simulink model "simpowersystems_simple_phasor_source"  (Simulink 8.1)
settings: Solver=FixedStepDiscrete  StartTime=0.0  StopTime=inf  FixedStep=1  MaxStep=1/60  RelTol=1e-3
InitFcn:
  | Ts = 1e-5;
undefined symbols (not defined in the file): j
libraries: powerlib x9, powerlib_extras x3, simulink x2
settings Model: Creator=sfrank1  LastModifiedBy=bjohnson

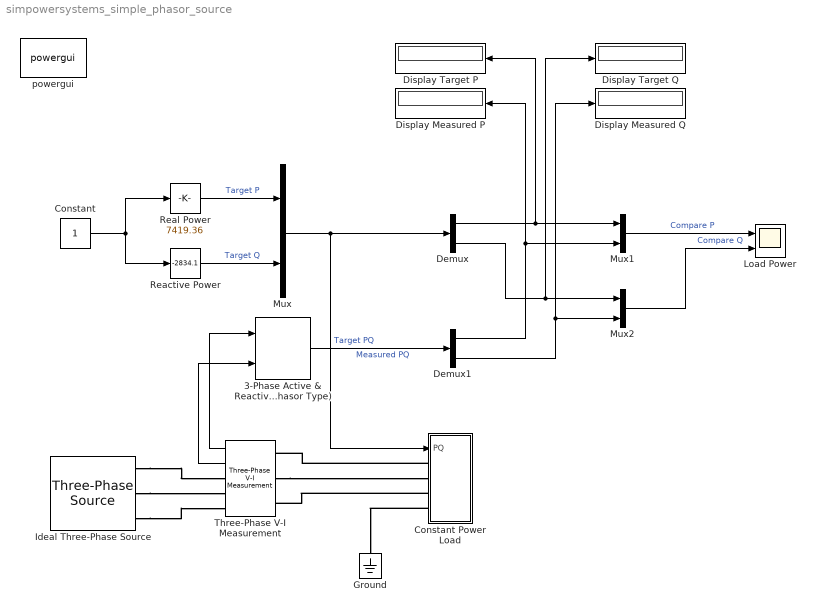
== system simpowersystems_simple_phasor_source ==
  3-Phase Active & Reactive Power (Phasor Type) : powerlib_extras/Phasor Library/3-Phase Active & Reactive Power (Phasor Type)
  Constant : Constant
  Constant Power Load : Subsystem  mask(Constant Power Load){VNom=480, fNom=60}
      mask prompts: VNom "Nominal line-to-line voltage (VRMS)"; fNom "Nominal frequency (Hz)"
      mask help: Implements a controllable constant power load, where VI* = P + jQ (in per-unit).
      mask Help: Implements a controllable constant power load, where VI* = P + jQ (in per-unit).
  Demux : Demux  Outputs=2
  Demux1 : Demux  Outputs=2
  Display Measured P : Display
  Display Measured Q : Display
  Display Target P : Display
  Display Target Q : Display
  Ground : powerlib/Elements/Ground  LConnTagsString=a
  Ideal Three-Phase Source : powerlib/Electrical Sources/Three-Phase Source  Voltage=480  PhaseAngle=0  Frequency=60  InternalConnection=Yg  SpecifyImpedance=on  Resistance=0  Inductance=0  ShortCircuitLevel=1e6  BaseVoltage=480  XRratio=1  BusType=swing  Pref=0  Qref=0  Qmin=-inf  Qmax=inf
  Load Power : Scope  NumInputPorts=2
      settings: TickLabels=on  YMin=7419.36~-2834.1  YMax=7419.36~-2834.1
  Mux : Mux  Inputs=2
  Mux1 : Mux  Inputs=2
  Mux2 : Mux  Inputs=2
  Reactive Power : simulink/Math Operations/Slider Gain  low=-5000  gain=-2834.1  high=5000
  Real Power : simulink/Math Operations/Slider Gain  low=0  gain=7419.36  high=10000
  Three-Phase V-I Measurement : powerlib/Measurements/Three-Phase V-I Measurement  VoltageMeasurement=phase-to-ground  SetLabelV=off  LabelV=Vabc  Vpu=off  VpuLL=off  CurrentMeasurement=yes  SetLabelI=off  LabelI=Iabc  Ipu=off  Pbase=100e6  Vbase=500e3  OutputType=Complex  PhasorSimulation=on  PSBequivalent=0
  powergui : powerlib/powergui  Priority=1  SimulationMode=Phasor  SolverType=Tustin  SampleTime=50e-6  frequency=60  SPID=off  DisableSnubberDevices=off  DisableRonSwitches=off  DisableVfSwitches=off  SwTol=0  Interpol=off  DisplayEquations=off  frequencyindice=60  Pbase=100e3  ErrMax=1e-4  Iterations=50  UnitsV=kV  UnitsW=MW  FunctionMessages=off  echomessages=off  HookPort=off  EnableUseOfTLC=off  x0status=blocks  RestoreLinks=warning  ResistiveCurrentMeasurement=off  Frange=[0:2:500]  Ylog=off  Xlog=on  ShowGrid=off  save=off  variable=ZData  ZoomFFT=off  StartTime=0.0  cycles=1  DisplayStyle=1  fundamental=60  FreqAxis=off  MaxFrequency=1000  frequencyindicesteady=1  RmsSteady=1  display=off  Ts=0  methode=off
  wires:
  Constant/1 -> Reactive Power/1, Real Power/1
  Real Power/1 -> Mux/1  "Target P"
  Mux/1 -> Constant Power Load/1(PQ), Demux/1  "Target PQ"
  Three-Phase V-I Measurement/1 -> 3-Phase Active & Reactive Power (Phasor Type)/1
  Three-Phase V-I Measurement/2 -> 3-Phase Active & Reactive Power (Phasor Type)/2
  Reactive Power/1 -> Mux/2  "Target Q"
  3-Phase Active & Reactive Power (Phasor Type)/1 -> Demux1/1  "Measured PQ"
  Mux1/1 -> Load Power/1  "Compare P"
  Mux2/1 -> Load Power/2  "Compare Q"
  Demux/1 -> Mux1/1, Display Target P/1
  Demux1/1 -> Display Measured P/1, Mux1/2
  Demux/2 -> Mux2/1, Display Target Q/1
  Demux1/2 -> Mux2/2, Display Measured Q/1
  connections:
  Constant Power Load/LConn3 -- Three-Phase V-I Measurement/LConn3
  Three-Phase V-I Measurement/LConn2 -- Constant Power Load/LConn2
  Constant Power Load/LConn1 -- Three-Phase V-I Measurement/LConn1
  Constant Power Load/LConn4 -- Ground/LConn1
  Ideal Three-Phase Source/RConn2 -- Three-Phase V-I Measurement/RConn2
  Ideal Three-Phase Source/RConn1 -- Three-Phase V-I Measurement/RConn1
  Ideal Three-Phase Source/RConn3 -- Three-Phase V-I Measurement/RConn3

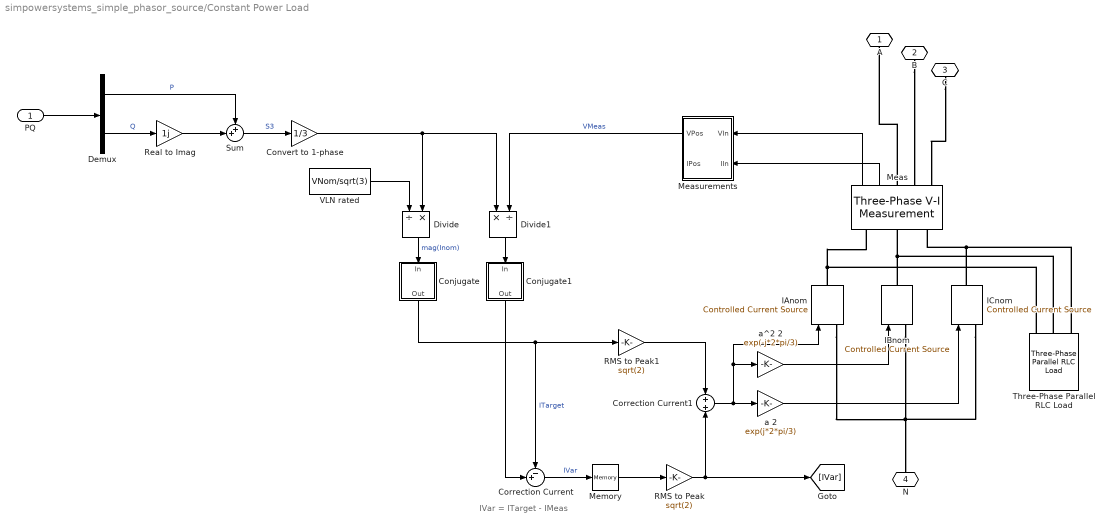
== system simpowersystems_simple_phasor_source/Constant Power Load ==
  note: IVar = ITarget - IMeas
  PQ : Inport  PortDimensions=2
  Conjugate : Subsystem
  Conjugate1 : Subsystem
  Convert to 1-phase : Gain  Gain=1/3
  Correction Current : Sum  Inputs=-+|
  Correction Current1 : Sum
  Demux : Demux  Outputs=2
  Divide : Product  Inputs=/*
  Divide1 : Product  Inputs=*/
  IAnom : powerlib/Electrical Sources/Controlled Current Source  Initialize=off  Source_Type=AC  Amplitude=0  Phase=0  Frequency=0  Measurements=Current
  IBnom : powerlib/Electrical Sources/Controlled Current Source  Initialize=off  Source_Type=AC  Amplitude=0  Phase=0  Frequency=0  Measurements=Current
  ICnom : powerlib/Electrical Sources/Controlled Current Source  Initialize=off  Source_Type=AC  Amplitude=0  Phase=0  Frequency=0  Measurements=Current
  Meas : powerlib/Measurements/Three-Phase V-I Measurement  VoltageMeasurement=phase-to-ground  SetLabelV=off  LabelV=Vabc  Vpu=off  VpuLL=off  CurrentMeasurement=yes  SetLabelI=off  LabelI=Iabc  Ipu=off  Pbase=100e6  Vbase=VNom  OutputType=Complex  PhasorSimulation=on  PSBequivalent=0
  Measurements : Subsystem
  Memory : Memory
  RMS to Peak : Gain  Gain=sqrt(2)
  RMS to Peak1 : Gain  Gain=sqrt(2)
  Real to Imag : Gain  Gain=1j
  Sum : Sum  Inputs=++|
  Three-Phase Parallel RLC Load : powerlib/Elements/Three-Phase Parallel RLC Load  LConnTagsString=A|B|C  Configuration=Y (grounded)  NominalVoltage=480  NominalFrequency=60  ActivePower=1e-9  InductivePower=0  CapacitivePower=0  Measurements=None  LoadType=constant Z
  VLN rated : Constant  Value=VNom/sqrt(3)
  a 2 : Gain  Gain=exp(j*2*pi/3)
  a^2 2 : Gain  Gain=exp(-j*2*pi/3)
  A : PMIOPort  Port=1  Side=Left
  B : PMIOPort  Port=2  Side=Left
  C : PMIOPort  Port=3  Side=Left
  N : PMIOPort  Port=4  Side=Left
  wires:
  PQ/1 -> Demux/1
  Demux/2 -> Real to Imag/1  "Q"
  Demux/1 -> Sum/1  "P"
  Real to Imag/1 -> Sum/2
  Sum/1 -> Convert to 1-phase/1  "S3"
  Convert to 1-phase/1 -> Divide/2, Divide1/1
  Divide/1 -> Conjugate/1(In)  "mag(Inom)"
  Correction Current/1 -> Memory/1  "IVar"
  Conjugate/1(Out) -> Correction Current/1, RMS to Peak1/1  "ITarget"
  RMS to Peak/1 -> [IVar], Correction Current1/2
  Memory/1 -> RMS to Peak/1
  VLN rated/1 -> Divide/1
  a 2/1 -> ICnom/1
  a^2 2/1 -> IBnom/1
  Meas/1 -> Measurements/1(VIn)
  Meas/2 -> Measurements/2(IIn)
  Measurements/1(VPos) -> Divide1/2  "VMeas"
  Divide1/1 -> Conjugate1/1(In)
  Conjugate1/1(Out) -> Correction Current/2
  Correction Current1/1 -> a^2 2/1, IAnom/1, a 2/1
  RMS to Peak1/1 -> Correction Current1/1
  connections:
  Meas/RConn1 -- A/RConn1
  B/RConn1 -- Meas/RConn2
  C/RConn1 -- Meas/RConn3
  IAnom/RConn1 -- Three-Phase Parallel RLC Load/LConn1 -- Meas/LConn1
  IBnom/RConn1 -- Three-Phase Parallel RLC Load/LConn2 -- Meas/LConn2
  ICnom/RConn1 -- Three-Phase Parallel RLC Load/LConn3 -- Meas/LConn3
  IBnom/LConn1 -- ICnom/LConn1 -- N/RConn1 -- IAnom/LConn1

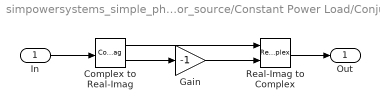
== system simpowersystems_simple_phasor_source/Constant Power Load/Conjugate ==
  In : Inport
  Complex to Real-Imag : ComplexToRealImag
  Gain : Gain  Gain=-1
  Real-Imag to Complex : RealImagToComplex
  Out : Outport
  wires:
  In/1 -> Complex to Real-Imag/1
  Complex to Real-Imag/1 -> Real-Imag to Complex/1
  Complex to Real-Imag/2 -> Gain/1
  Gain/1 -> Real-Imag to Complex/2
  Real-Imag to Complex/1 -> Out/1

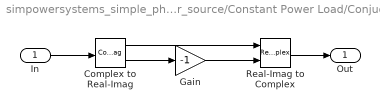
== system simpowersystems_simple_phasor_source/Constant Power Load/Conjugate1 ==
  In : Inport
  Complex to Real-Imag : ComplexToRealImag
  Gain : Gain  Gain=-1
  Real-Imag to Complex : RealImagToComplex
  Out : Outport
  wires:
  Real-Imag to Complex/1 -> Out/1
  Gain/1 -> Real-Imag to Complex/2
  Complex to Real-Imag/2 -> Gain/1
  Complex to Real-Imag/1 -> Real-Imag to Complex/1
  In/1 -> Complex to Real-Imag/1

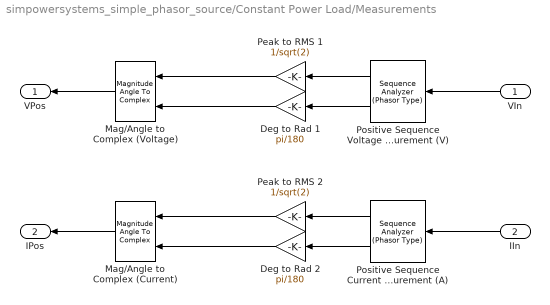
== system simpowersystems_simple_phasor_source/Constant Power Load/Measurements ==
  VIn : Inport
  IIn : Inport  Port=2
  Deg to Rad 1 : Gain  Gain=pi/180
  Deg to Rad 2 : Gain  Gain=pi/180
  Mag/Angle to Complex (Current) : MagnitudeAngleToComplex
  Mag/Angle to Complex (Voltage) : MagnitudeAngleToComplex
  Peak to RMS 1 : Gain  Gain=1/sqrt(2)
  Peak to RMS 2 : Gain  Gain=1/sqrt(2)
  Positive Sequence Current Measurement (A) : powerlib_extras/Phasor Library/Sequence Analyzer (Phasor Type)  seq=Positive
  Positive Sequence Voltage Measurement (V) : powerlib_extras/Phasor Library/Sequence Analyzer (Phasor Type)  seq=Positive
  VPos : Outport
  IPos : Outport  Port=2
  wires:
  Positive Sequence Voltage Measurement (V)/1 -> Peak to RMS 1/1
  Positive Sequence Current Measurement (A)/1 -> Peak to RMS 2/1
  Positive Sequence Current Measurement (A)/2 -> Deg to Rad 2/1
  Peak to RMS 1/1 -> Mag/Angle to Complex (Voltage)/1
  VIn/1 -> Positive Sequence Voltage Measurement (V)/1
  IIn/1 -> Positive Sequence Current Measurement (A)/1
  Mag/Angle to Complex (Voltage)/1 -> VPos/1
  Mag/Angle to Complex (Current)/1 -> IPos/1
  Peak to RMS 2/1 -> Mag/Angle to Complex (Current)/1
  Deg to Rad 1/1 -> Mag/Angle to Complex (Voltage)/2
  Positive Sequence Voltage Measurement (V)/2 -> Deg to Rad 1/1
  Deg to Rad 2/1 -> Mag/Angle to Complex (Current)/2
